simulink model "allModes"  (R2019a)
settings: Solver=FixedStepAuto  StartTime=0.0  StopTime=inf  FixedStep=1/1000  RelTol=1e-3  EnableMultiTasking=on
undefined symbols (not defined in the file or in its folder): D0, D1, D10, D11, D12, D13, D2, D3, D4, D5, D6, D7, D8, D9, PTA0, PTA1, PTA2, PTB23, PTB9, PTC16, PTC17, PTC2, PTC3, PTC4, PTD0, PTD1, PTD2, PTD3
libraries: frdmk64flib x16
settings Model: ExtModeTrigDuration=5  OrderedModelArguments=off  Creator=adrso  LastModifiedBy=adrso
settings OptimizationCC: EnhancedBackFolding=on  PassReuseOutputArgsAs=Individual arguments  MaxStackSize=64  OptimizeBlockOrder=speed  DifferentSizesBufferReuse=on  OptimizationCustomize=off
settings DebuggingCC: ParameterTunabilityLossMsg=error
settings HardwareCC: ProdBitPerPointer=32  ProdBitPerSizeT=32  ProdBitPerPtrDiffT=32  ProdLargestAtomicInteger=Long  ProdLargestAtomicFloat=Double  ProdWordSize=32  ProdHWDeviceType=ARM Compatible->ARM Cortex
settings SFSimCC: MATLABDynamicMemAlloc=off
settings RTWCC: SystemTargetFile=ert.tlc  HardwareBoard=NXP FRDM-K64F  TLCOptions="-aInlineSetEventsForThisBaseRateFcn=TLC_FALSE -aSuppressMultiTaskScheduler=TLC_FALSE  -aRateBasedStepFcn=0"  TemplateMakefile=ert_default_tmf  GenerateReport=on  Toolchain=GNU Tools for ARM Embedded Processors  IncludeHyperlinkInReport=on  LaunchReport=on  GenerateTraceInfo=on  GenerateTraceReport=on  GenerateTraceReportSl=on  GenerateTraceReportSf=on  GenerateTraceReportEml=on
settings CodeAppCC: ForceParamTrailComments=on  IgnoreCustomStorageClasses=off  OperatorAnnotations=on  SimulinkDataObjDesc=on  SFDataObjDesc=on  InsertBlockDesc=on

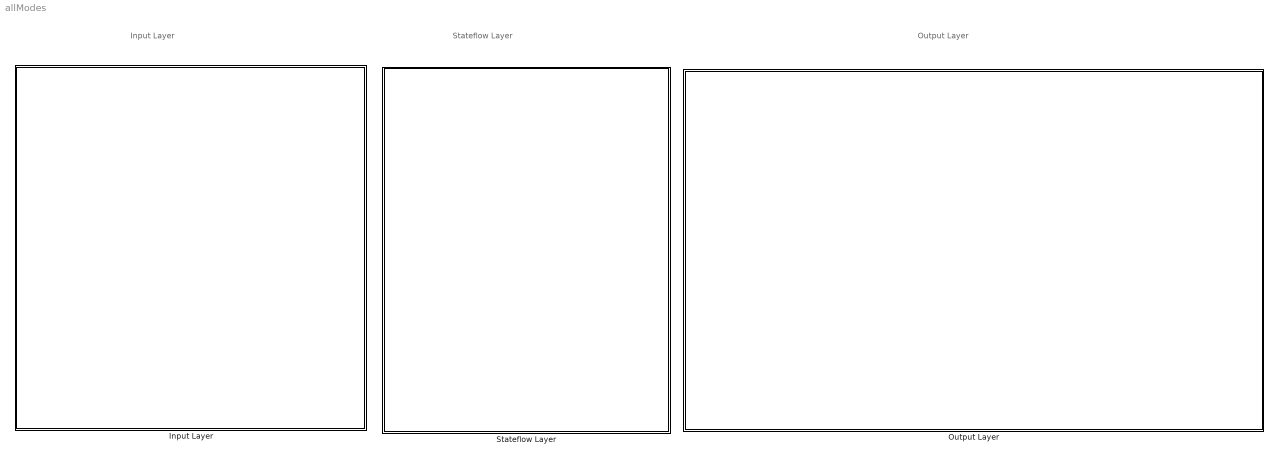
== system allModes ==
  note: Input Layer
  note: Stateflow Layer
  note: Output Layer
  Input Layer : Subsystem
      mask Display: image('pacemakerInChest.jpg');
  Output Layer : Subsystem
      mask Display: image('frdmk64f.jpg');
  Stateflow Layer : Subsystem
      mask Display: image('matlabMeme.png');

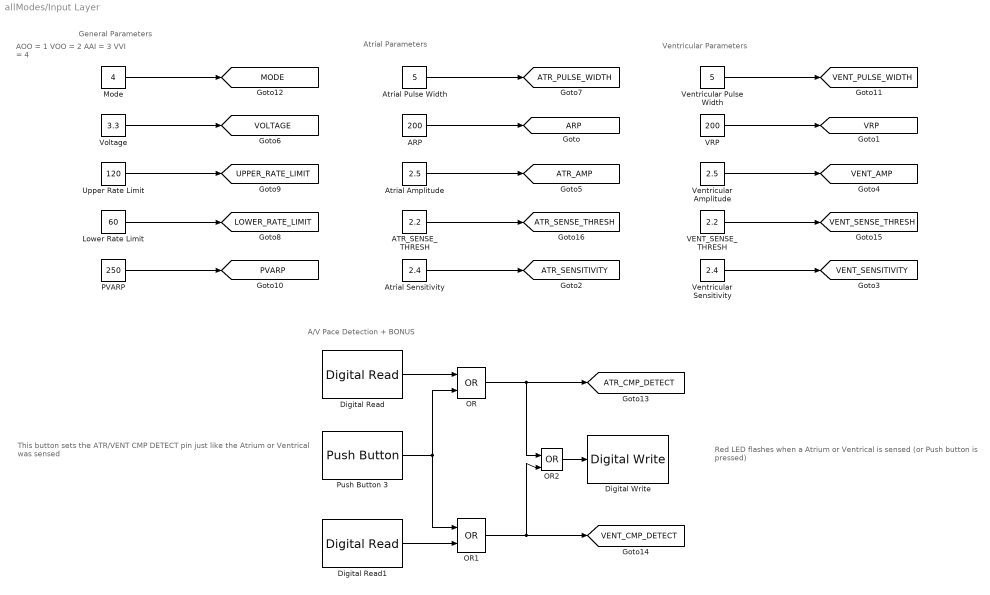
== system allModes/Input Layer ==
  note: AOO = 1
      | VOO = 2
      | AAI = 3
      | VVI = 4
  note: Red LED flashes when a Atrium or Ventrical
      | is sensed (or Push button is pressed)
  note: This button sets the ATR/VENT CMP DETECT
      | pin just like the Atrium or Ventrical was sensed
  note: Ventricular Parameters
  note: Atrial Parameters
  note: A/V Pace Detection + BONUS
  note: General Parameters
  ARP : Constant  Value=200  OutDataTypeStr=uint16
  ATR_SENSE_THRESH : Constant  Value=2.2  OutDataTypeStr=double
  Atrial Amplitude : Constant  Value=2.5  OutDataTypeStr=double
  Atrial Pulse Width : Constant  Value=5  OutDataTypeStr=uint8
  Atrial Sensitivity : Constant  Value=2.4  OutDataTypeStr=double
  Digital Read : frdmk64flib/Digital Read  Whichpin=PTC16 (D0)  SampleTime=-1
      settings: SourceProductName=Simulink Coder Support Package for NXP FRDM-K64F Board
  Digital Read1 : frdmk64flib/Digital Read  Whichpin=PTC17 (D1)  SampleTime=-1
      settings: SourceProductName=Simulink Coder Support Package for NXP FRDM-K64F Board
  Digital Write : frdmk64flib/Digital Write  Whichpin=RED_LED
      settings: SourceProductName=Simulink Coder Support Package for NXP FRDM-K64F Board
  Lower Rate Limit : Constant  Value=60  OutDataTypeStr=uint8
  Mode : Constant  Value=4  OutDataTypeStr=uint8
  OR : Logic  Operator=OR  IconShape=distinctive  AllPortsSameDT=off  OutDataTypeStr=boolean
  OR1 : Logic  Operator=OR  IconShape=distinctive  AllPortsSameDT=off  OutDataTypeStr=boolean
  OR2 : Logic  Operator=OR  IconShape=distinctive  AllPortsSameDT=off  OutDataTypeStr=boolean
  PVARP : Constant  Value=250  OutDataTypeStr=uint16
  Push Button 3 : frdmk64flib/Push Button  Whichswitch=SW3  SampleTime1=-1
      settings: SourceProductName=Simulink Coder Support Package for NXP FRDM-K64F Board
  Upper Rate Limit : Constant  Value=120  OutDataTypeStr=uint8
  VENT_SENSE_THRESH : Constant  Value=2.2  OutDataTypeStr=double
  VRP : Constant  Value=200  OutDataTypeStr=uint16
  Ventricular Amplitude : Constant  Value=2.5  OutDataTypeStr=double
  Ventricular Pulse Width : Constant  Value=5  OutDataTypeStr=uint8
  Ventricular Sensitivity : Constant  Value=2.4  OutDataTypeStr=double
  Voltage : Constant  Value=3.3  OutDataTypeStr=double
  tag scope: ARP=global, ATR_AMP=global, ATR_CMP_DETECT=global, ATR_PULSE_WIDTH=global, ATR_SENSE_THRESH=global, ATR_SENSITIVITY=global, LOWER_RATE_LIMIT=global, MODE=global, PVARP=global, UPPER_RATE_LIMIT=global, VENT_AMP=global, VENT_CMP_DETECT=global, VENT_PULSE_WIDTH=global, VENT_SENSE_THRESH=global, VENT_SENSITIVITY=global, VOLTAGE=global, VRP=global
  wires:
  Ventricular Amplitude/1 -> [VENT_AMP]
  ARP/1 -> [ARP]
  Atrial Amplitude/1 -> [ATR_AMP]
  VRP/1 -> [VRP]
  Voltage/1 -> [VOLTAGE]
  Atrial Sensitivity/1 -> [ATR_SENSITIVITY]
  Ventricular Sensitivity/1 -> [VENT_SENSITIVITY]
  Upper Rate Limit/1 -> [UPPER_RATE_LIMIT]
  Mode/1 -> [MODE]
  Lower Rate Limit/1 -> [LOWER_RATE_LIMIT]
  Ventricular Pulse Width/1 -> [VENT_PULSE_WIDTH]
  Atrial Pulse Width/1 -> [ATR_PULSE_WIDTH]
  Digital Read1/1 -> OR1/2
  VENT_SENSE_THRESH/1 -> [VENT_SENSE_THRESH]
  ATR_SENSE_THRESH/1 -> [ATR_SENSE_THRESH]
  OR/1 -> OR2/1, [ATR_CMP_DETECT]
  Digital Read/1 -> OR/1
  Push Button 3/1 -> OR/2, OR1/1
  OR1/1 -> OR2/2, [VENT_CMP_DETECT]
  OR2/1 -> Digital Write/1
  PVARP/1 -> [PVARP]

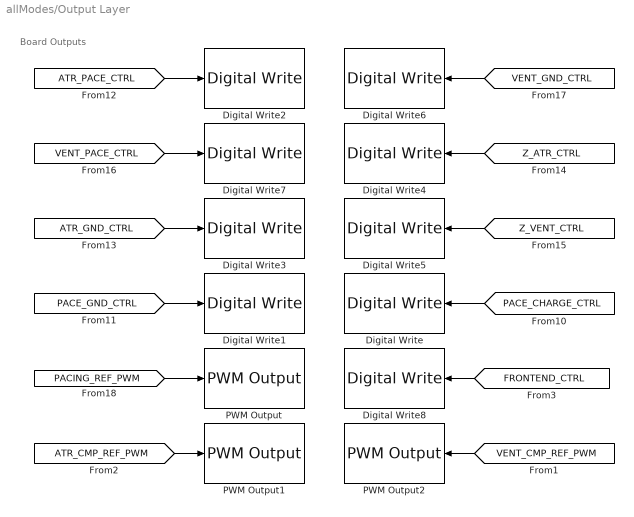
== system allModes/Output Layer ==
  note: Board Outputs
  Digital Write : frdmk64flib/Digital Write  Whichpin=PTB9 (D2)
      settings: SourceProductName=Simulink Coder Support Package for NXP FRDM-K64F Board
  Digital Write1 : frdmk64flib/Digital Write  Whichpin=PTD0 (D10)
      settings: SourceProductName=Simulink Coder Support Package for NXP FRDM-K64F Board
  Digital Write2 : frdmk64flib/Digital Write  Whichpin=PTA0 (D8)
      settings: SourceProductName=Simulink Coder Support Package for NXP FRDM-K64F Board
  Digital Write3 : frdmk64flib/Digital Write  Whichpin=PTD2 (D11)
      settings: SourceProductName=Simulink Coder Support Package for NXP FRDM-K64F Board
  Digital Write4 : frdmk64flib/Digital Write  Whichpin=PTB23 (D4)
      settings: SourceProductName=Simulink Coder Support Package for NXP FRDM-K64F Board
  Digital Write5 : frdmk64flib/Digital Write  Whichpin=PTC3 (D7)
      settings: SourceProductName=Simulink Coder Support Package for NXP FRDM-K64F Board
  Digital Write6 : frdmk64flib/Digital Write  Whichpin=PTD3 (D12)
      settings: SourceProductName=Simulink Coder Support Package for NXP FRDM-K64F Board
  Digital Write7 : frdmk64flib/Digital Write  Whichpin=PTC4 (D9)
      settings: SourceProductName=Simulink Coder Support Package for NXP FRDM-K64F Board
  Digital Write8 : frdmk64flib/Digital Write  Whichpin=PTD1 (D13)
      settings: SourceProductName=Simulink Coder Support Package for NXP FRDM-K64F Board
  PWM Output : frdmk64flib/PWM Output  Whichpin=PTA2 (D5)  InitialFrequency=2000  InitialDutyCycle=30
      settings: SourceProductName=Simulink Coder Support Package for NXP FRDM-K64F Board
  PWM Output1 : frdmk64flib/PWM Output  Whichpin=PTC2 (D6)  InitialFrequency=2000  InitialDutyCycle=30
      settings: SourceProductName=Simulink Coder Support Package for NXP FRDM-K64F Board
  PWM Output2 : frdmk64flib/PWM Output  Whichpin=PTA1 (D3)  InitialFrequency=2000  InitialDutyCycle=30
      settings: SourceProductName=Simulink Coder Support Package for NXP FRDM-K64F Board
  wires:
  [PACING_REF_PWM] -> PWM Output/1
  [VENT_GND_CTRL] -> Digital Write6/1
  [ATR_GND_CTRL] -> Digital Write3/1
  [VENT_PACE_CTRL] -> Digital Write7/1
  [PACE_CHARGE_CTRL] -> Digital Write/1
  [ATR_PACE_CTRL] -> Digital Write2/1
  [Z_VENT_CTRL] -> Digital Write5/1
  [Z_ATR_CTRL] -> Digital Write4/1
  [PACE_GND_CTRL] -> Digital Write1/1
  [ATR_CMP_REF_PWM] -> PWM Output1/1
  [VENT_CMP_REF_PWM] -> PWM Output2/1
  [FRONTEND_CTRL] -> Digital Write8/1

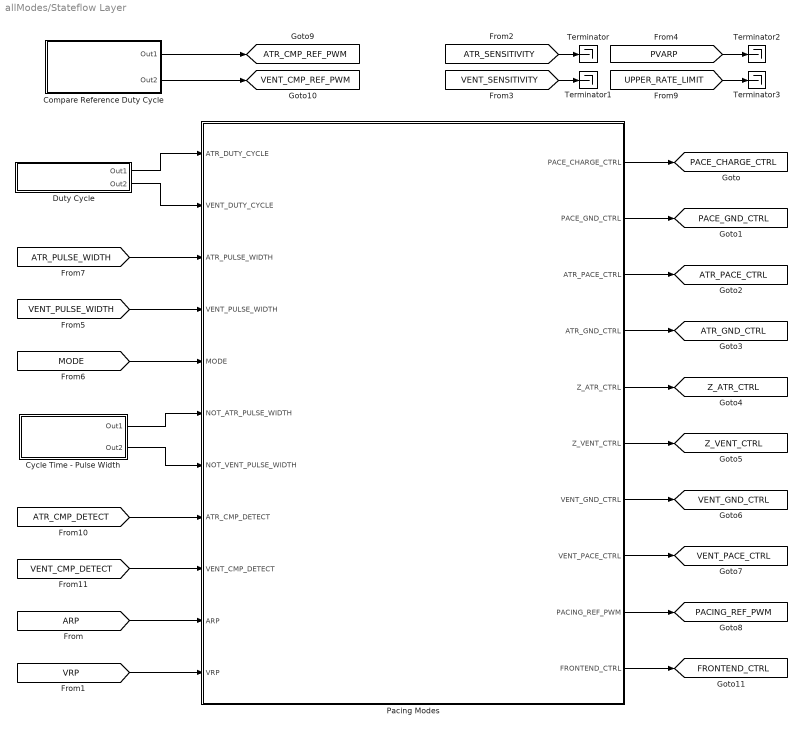
== system allModes/Stateflow Layer ==
  Compare Reference Duty Cycle : Subsystem
  Cycle Time - Pulse Width : Subsystem
  Duty Cycle : Subsystem
  Pacing Modes : Stateflow chart  BlockKeywords=__PRM__SERIALIZED__DATA__:Stateflow Chart,Stateflow Diagram  TreatAsAtomicUnit=on
  Terminator{,1..3} (4 alike) : Terminator
  tag scope: ATR_CMP_REF_PWM=global, ATR_GND_CTRL=global, ATR_PACE_CTRL=global, FRONTEND_CTRL=global, PACE_CHARGE_CTRL=global, PACE_GND_CTRL=global, PACING_REF_PWM=global, VENT_CMP_REF_PWM=global, VENT_GND_CTRL=global, VENT_PACE_CTRL=global, Z_ATR_CTRL=global, Z_VENT_CTRL=global
  wires:
  [ATR_PULSE_WIDTH] -> Pacing Modes/3(ATR_PULSE_WIDTH)
  [VENT_PULSE_WIDTH] -> Pacing Modes/4(VENT_PULSE_WIDTH)
  Duty Cycle/1(Out1) -> Pacing Modes/1(ATR_DUTY_CYCLE)
  Duty Cycle/2(Out2) -> Pacing Modes/2(VENT_DUTY_CYCLE)
  Pacing Modes/6(Z_VENT_CTRL) -> [Z_VENT_CTRL]
  Pacing Modes/8(VENT_PACE_CTRL) -> [VENT_PACE_CTRL]
  Pacing Modes/4(ATR_GND_CTRL) -> [ATR_GND_CTRL]
  Pacing Modes/3(ATR_PACE_CTRL) -> [ATR_PACE_CTRL]
  Pacing Modes/9(PACING_REF_PWM) -> [PACING_REF_PWM]
  Pacing Modes/2(PACE_GND_CTRL) -> [PACE_GND_CTRL]
  Pacing Modes/1(PACE_CHARGE_CTRL) -> [PACE_CHARGE_CTRL]
  Pacing Modes/5(Z_ATR_CTRL) -> [Z_ATR_CTRL]
  Pacing Modes/7(VENT_GND_CTRL) -> [VENT_GND_CTRL]
  [MODE] -> Pacing Modes/5(MODE)
  Cycle Time - Pulse Width/1(Out1) -> Pacing Modes/6(NOT_ATR_PULSE_WIDTH)
  Cycle Time - Pulse Width/2(Out2) -> Pacing Modes/7(NOT_VENT_PULSE_WIDTH)
  [VENT_CMP_DETECT] -> Pacing Modes/9(VENT_CMP_DETECT)
  [ATR_CMP_DETECT] -> Pacing Modes/8(ATR_CMP_DETECT)
  Pacing Modes/10(FRONTEND_CTRL) -> [FRONTEND_CTRL]
  [ARP] -> Pacing Modes/10(ARP)
  [VRP] -> Pacing Modes/11(VRP)
  Compare Reference Duty Cycle/1(Out1) -> [ATR_CMP_REF_PWM]
  Compare Reference Duty Cycle/2(Out2) -> [VENT_CMP_REF_PWM]
  [ATR_SENSITIVITY] -> Terminator/1
  [VENT_SENSITIVITY] -> Terminator1/1
  [UPPER_RATE_LIMIT] -> Terminator3/1
  [PVARP] -> Terminator2/1

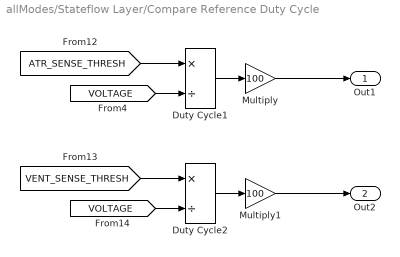
== system allModes/Stateflow Layer/Compare Reference Duty Cycle ==
  Duty Cycle1 : Product  Inputs=*/
  Duty Cycle2 : Product  Inputs=*/
  Multiply : Gain  Gain=100
  Multiply1 : Gain  Gain=100
  Out1 : Outport
  Out2 : Outport  Port=2
  wires:
  Multiply1/1 -> Out2/1
  [VENT_SENSE_THRESH] -> Duty Cycle2/1
  [VOLTAGE] -> Duty Cycle1/2
  [VOLTAGE] -> Duty Cycle2/2
  Duty Cycle2/1 -> Multiply1/1
  [ATR_SENSE_THRESH] -> Duty Cycle1/1
  Duty Cycle1/1 -> Multiply/1
  Multiply/1 -> Out1/1

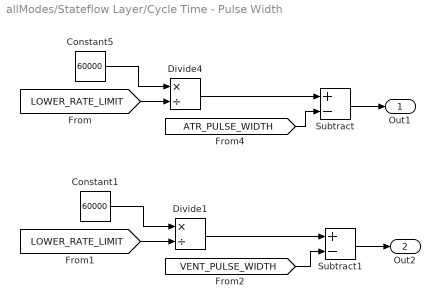
== system allModes/Stateflow Layer/Cycle Time - Pulse Width ==
  Constant1 : Constant  Value=60000
  Constant5 : Constant  Value=60000
  Divide1 : Product  Inputs=*/  RndMeth=Nearest
  Divide4 : Product  Inputs=*/  RndMeth=Nearest
  Subtract : Sum  Inputs=+-  OutDataTypeStr=uint16  RndMeth=Nearest
  Subtract1 : Sum  Inputs=+-  OutDataTypeStr=uint16  RndMeth=Nearest
  Out1 : Outport
  Out2 : Outport  Port=2
  wires:
  [LOWER_RATE_LIMIT] -> Divide4/2
  Constant5/1 -> Divide4/1
  Divide4/1 -> Subtract/1
  [ATR_PULSE_WIDTH] -> Subtract/2
  Subtract/1 -> Out1/1
  Divide1/1 -> Subtract1/1
  Constant1/1 -> Divide1/1
  [LOWER_RATE_LIMIT] -> Divide1/2
  Subtract1/1 -> Out2/1
  [VENT_PULSE_WIDTH] -> Subtract1/2

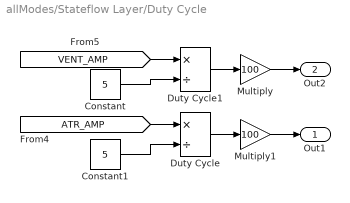
== system allModes/Stateflow Layer/Duty Cycle ==
  Constant : Constant  Value=5  OutDataTypeStr=double
  Constant1 : Constant  Value=5  OutDataTypeStr=double
  Duty Cycle : Product  Inputs=*/
  Duty Cycle1 : Product  Inputs=*/
  Multiply : Gain  Gain=100
  Multiply1 : Gain  Gain=100
  Out1 : Outport
  Out2 : Outport  Port=2
  wires:
  Constant1/1 -> Duty Cycle/2
  [ATR_AMP] -> Duty Cycle/1
  Constant/1 -> Duty Cycle1/2
  [VENT_AMP] -> Duty Cycle1/1
  Duty Cycle1/1 -> Multiply/1
  Multiply/1 -> Out2/1
  Multiply1/1 -> Out1/1
  Duty Cycle/1 -> Multiply1/1

== stateflow chart allModes/Stateflow Layer/Pacing Modes ==
  state AAI [group]
    state INTERMIDIATE
      during:
      %Discharge C21
      PACE_GND_CTRL = true
      VENT_PACE_CTRL = false
      Z_ATR_CTRL = false
      Z_VENT_CTRL = false
      ATR_PACE_CTRL = false
      ATR_GND_CTRL = true
      VENT_GND_CTRL = false
      %Charge C22
      ATR_PACE_CTRL = false
      VENT_PACE_CTRL = false
      PACING_REF_PWM = ATR_DUTY_CYCLE
      PACE_CHARGE_CTRL = true
    state CHARGING
      during:
      %Charge C22
      ATR_PACE_CTRL = false
      VENT_PACE_CTRL = false
      PACING_REF_PWM = ATR_DUTY_CYCLE
      PACE_CHARGE_CTRL = true
      %Discharge C21
      PACE_GND_CTRL = true
      VENT_PACE_CTRL = false
      Z_ATR_CTRL = false
      Z_VENT_CTRL = false
      ATR_PACE_CTRL = false
      ATR_GND_CTRL = true
      VENT_GND_CTRL = false
    state DISCHARGING
      during:
      %Discharge C22 into ATR
      %Charge C21
      PACE_CHARGE_CTRL = false
      PACE_GND_CTRL = true
      ATR_PACE_CTRL = true
      ATR_GND_CTRL = false
      Z_ATR_CTRL = false
      Z_VENT_CTRL = false
      VENT_GND_CTRL = false
      VENT_PACE_CTRL = false
    AAI.CHARGING -> AAI.INTERMIDIATE [order 2] : [ATR_CMP_DETECT == true]
    AAI.DISCHARGING -> AAI.INTERMIDIATE : after(ATR_PULSE_WIDTH, msec)
    AAI.INTERMIDIATE -> AAI.CHARGING : after(ARP, msec)
    AAI.CHARGING -> AAI.DISCHARGING [order 1] : after(NOT_ATR_PULSE_WIDTH - ARP, msec)
  state AOO [group]
    state CHARGING
      during:
      %Charge C22
      ATR_PACE_CTRL = false
      VENT_PACE_CTRL = false
      PACING_REF_PWM = ATR_DUTY_CYCLE
      PACE_CHARGE_CTRL = true
      %Discharge C21
      PACE_GND_CTRL = true
      VENT_PACE_CTRL = false
      Z_ATR_CTRL = false
      Z_VENT_CTRL = false
      ATR_PACE_CTRL = false
      ATR_GND_CTRL = true
      VENT_GND_CTRL = false
    state DISCHARGING
      during:
      %Discharge C22 into ATR
      %Charge C21
      PACE_CHARGE_CTRL = false
      PACE_GND_CTRL = true
      ATR_PACE_CTRL = true
      ATR_GND_CTRL = false
      Z_ATR_CTRL = false
      Z_VENT_CTRL = false
      VENT_GND_CTRL = false
      VENT_PACE_CTRL = false
    AOO.CHARGING -> AOO.DISCHARGING [order 1] : after(NOT_ATR_PULSE_WIDTH, msec)
    AOO.DISCHARGING -> AOO.CHARGING : after(ATR_PULSE_WIDTH,msec)
  state Start
  state VOO [group]
    state DISCHARGING
      during:
      %Discharge C22 into VENT
      %Charge C21
      PACE_CHARGE_CTRL = false
      PACE_GND_CTRL = true
      ATR_PACE_CTRL = false
      ATR_GND_CTRL = false
      Z_ATR_CTRL = false
      Z_VENT_CTRL = false
      VENT_GND_CTRL = false
      VENT_PACE_CTRL = true
    state CHARGING
      during:
      %Charge C22
      ATR_PACE_CTRL = false
      VENT_PACE_CTRL = false
      PACING_REF_PWM = VENT_DUTY_CYCLE
      PACE_CHARGE_CTRL = true
      %Discharge C21
      PACE_GND_CTRL = true
      VENT_PACE_CTRL = false
      Z_ATR_CTRL = false
      Z_VENT_CTRL = false
      ATR_PACE_CTRL = false
      ATR_GND_CTRL = false
      VENT_GND_CTRL = true
    VOO.CHARGING -> VOO.DISCHARGING [order 1] : after(NOT_VENT_PULSE_WIDTH,msec)
    VOO.DISCHARGING -> VOO.CHARGING : after(VENT_PULSE_WIDTH,msec)
  state VVI [group]
    state INTERMIDIATE
      during:
      %Discharge C21
      PACE_GND_CTRL = true
      VENT_PACE_CTRL = false
      Z_ATR_CTRL = false
      Z_VENT_CTRL = false
      ATR_PACE_CTRL = false
      ATR_GND_CTRL = false
      VENT_GND_CTRL = true
      %Charge C22
      ATR_PACE_CTRL = false
      VENT_PACE_CTRL = false
      PACING_REF_PWM = VENT_DUTY_CYCLE
      PACE_CHARGE_CTRL = true
    state DISCHARGING
      during:
      %Discharge C22 into VENT
      %Charge C21
      PACE_CHARGE_CTRL = false
      PACE_GND_CTRL = true
      ATR_PACE_CTRL = false
      ATR_GND_CTRL = false
      Z_ATR_CTRL = false
      Z_VENT_CTRL = false
      VENT_GND_CTRL = false
      VENT_PACE_CTRL = true
    state CHARGING
      during:
      %Charge C22
      ATR_PACE_CTRL = false
      VENT_PACE_CTRL = false
      PACING_REF_PWM = VENT_DUTY_CYCLE
      PACE_CHARGE_CTRL = true
      %Discharge C21
      PACE_GND_CTRL = true
      VENT_PACE_CTRL = false
      Z_ATR_CTRL = false
      Z_VENT_CTRL = false
      ATR_PACE_CTRL = false
      ATR_GND_CTRL = false
      VENT_GND_CTRL = true
    VVI.CHARGING -> VVI.INTERMIDIATE [order 1] : [VENT_CMP_DETECT == true]
    VVI.DISCHARGING -> VVI.INTERMIDIATE : after(VENT_PULSE_WIDTH, msec)
    VVI.INTERMIDIATE -> VVI.CHARGING : after(VRP, msec)
    VVI.CHARGING -> VVI.DISCHARGING [order 2] : after(NOT_VENT_PULSE_WIDTH-VRP, msec)
  VOO.CHARGING -> Start [order 2] : [MODE ~= 2]
  AOO.CHARGING -> Start [order 2] : [MODE ~= 1]
  AAI.CHARGING -> Start [order 3] : [MODE ~= 3]
  VVI.CHARGING -> Start [order 3] : [MODE ~= 4]
  Start -> AAI.CHARGING [order 4] : [MODE == 3]
  Start -> AOO.CHARGING [order 1] : [MODE == 1]
  Start -> VVI.CHARGING [order 3] : [MODE == 4]
  Start -> VOO.CHARGING [order 2] : [MODE == 2]
  (default) -> Start
  data: ATR_DUTY_CYCLE input double; VENT_DUTY_CYCLE input double; ATR_PULSE_WIDTH input uint8; PACE_CHARGE_CTRL output boolean; PACE_GND_CTRL output boolean; ATR_PACE_CTRL output boolean; ATR_GND_CTRL output boolean; Z_ATR_CTRL output boolean =false; Z_VENT_CTRL output boolean =false; VENT_GND_CTRL output boolean; VENT_PACE_CTRL output boolean; PACING_REF_PWM output double; VENT_PULSE_WIDTH input uint8; MODE input uint8; NOT_ATR_PULSE_WIDTH input uint16; NOT_VENT_PULSE_WIDTH input uint16; ATR_CMP_DETECT input boolean; VENT_CMP_DETECT input boolean; FRONTEND_CTRL output boolean =true; ARP input uint16; VRP input uint16
